simulink model "ProjectRem"  (R2025b)
settings: Solver=VariableStepAuto  StartTime=0.0  StopTime=80  RelTol=1e-3
libraries: deeplib x1
settings Model: Creator=ilaga  LastModifiedBy=ilaga

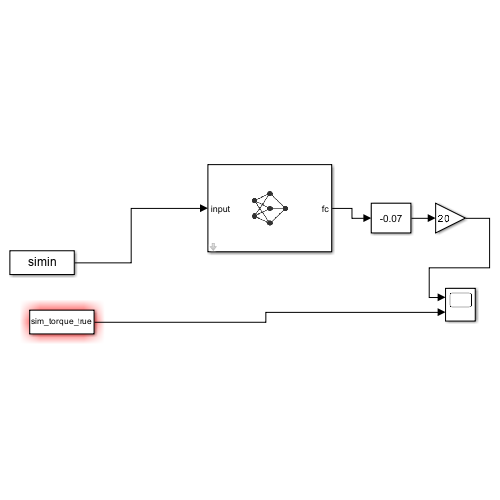
[thumbnail: Simulink's stored preview of the top-level diagram]
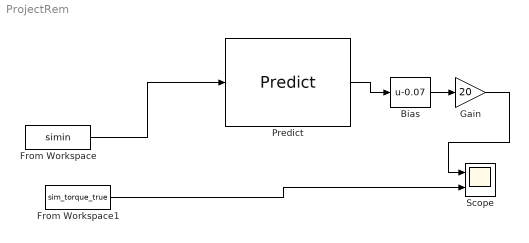
== system ProjectRem ==
  Bias : Bias  Bias=-0.07  SaturateOnIntegerOverflow=off
  From Workspace : FromWorkspace  VariableName=simin  SampleTime=0.01
  From Workspace1 : FromWorkspace  VariableName=sim_torque_true
  Gain : Gain  Gain=20
  Predict : deeplib/Predict  Network=Network from MAT-file  NetworkFunction=squeezenet  NetworkFilePath=C:\Users\ilaga\Documents\Wesa\torque_lstm_model.mat  MiniBatchSize=1  InputDataFormats={'input', 'TCB';}  Predictions=on  Activations={}  ForceInterpretedSim=off  EnableDLNetwork=on  LastKnownNetworkFilePath='C:\Users\ilaga\Documents\Wesa\torque_lstm_model.mat'  LastKnownNetworkTimeStamp=740100.863842592574656009674072265625
  Scope : Scope  NumInputPorts=2
      settings: ActiveDisplayYMinimum=-2.0568652260061748  ActiveDisplayYMaximum=1.5713355080367362
  wires:
  Predict/1 -> Bias/1
  From Workspace/1 -> Predict/1
  Gain/1 -> Scope/1
  Bias/1 -> Gain/1
  From Workspace1/1 -> Scope/2
